simulink model "ATRIAS_vnmc"  (R2015a)
settings: Solver=ode45  StartTime=0.0  StopTime=60  FixedStep=1e-3  MinStep=1e-6  RelTol=1e-3  AbsTol=1e-4
values from neighbouring files (symbols this model uses):
  initial_boom_yaw = initial_boom_yaw + delta_yaw0    [run_model.m]
  max_floor_diff = cost_fun_opts.max_floor_diff    [opt_cmaes.m]    (also in run_model.m; set_all_params_simple.m = 0)
  noise_on_off = cost_fun_opts.noise_on_off    [opt_cmaes.m]    (also in run_model.m; set_all_params_simple.m = 0)
  noise_seed = cost_fun_opts.noise_seed    [opt_cmaes.m]    (also in run_model.m; set_all_params_simple.m = 1)
  noise_variance = cost_fun_opts.noise_variance    [opt_cmaes.m]    (also in run_model.m; set_all_params_simple.m = 0.000174532925199)
  SEA_swing_ctrl_on_off = cost_fun_opts.SEA_swing_ctrl_on_off    [opt_cmaes.m]    (also in run_model.m; set_all_params_simple.m = 0)
  sim_t = simout.twalk    [run_model.m]
  steady_dist = cost_fun_opts.steady_dist    [opt_cmaes.m]    (also in run_model.m; set_all_params_simple.m = 10)
  ts_anim = 0.0333    [run_model.m]
undefined symbols (not defined in the file or in its folder): A1_notch_f1, A2_notch_f1, A_lpf_dtau, A_lpf_velocity, B1_lpf_dtau, B1_lpf_velocity, B1_notch_f1, B2_lpf_dtau, B2_lpf_velocity, B2_notch_f1, b_hmotor, b_leg_spring, b_rotor, base_color_d, boom_color_d, boom_mount_to_center_diagonal, breakaway_friction, c, c_jointstop, com_height_offset, contactThr, coulomb_friction, CtrlPar_theta0, D12_S, D12_T, d_com, ddx_max, ddy_max, delta_phi_max, delta_phi_max_buffer, delta_phi_max_dropoff, delta_phi_min, des_forward_velocity, DS_width, dtau_des_max, dtheta0_vmc, dx0_vmc, dy_max, eref, fblink_color_d, fcut_acceleration, floor_color_d, floor_tile_width, floor_zero_height, FmaxBFSH, FmaxGLU, FmaxHAM, FmaxHFL, FmaxRF, FmaxVAS, FPCtrlPar, friction_linear_zone, g, gain_nodes_sea_torque, gamma_stance_thr, gamma_swing_thr, hip_height, HIP_MTR_MAX_CONT_TORQUE, HIP_MTR_MAX_TORQUE, hshaft_color_d ... (+236)
libraries: sm_lib x280, nesl_utility x174, simulink x114, simulink_extras x58, fl_lib x16, mblibv1 x2, dspswit3 x2
(part 12 of 23)

== system ATRIAS_vnmc/atrias_system/Ground Contact/R Contact/3D Contact ==
  RefPt [m m m] : Inport
  nVec [m m m] : Inport  Port=2
  pVec [m m m] : Inport  Port=3
  vVec [m/s m/s m/s] : Inport  Port=4
  Contact! : EnablePort  StatesWhenEnabling=reset
  Friction Switch : Subsystem
  Kinetic Friction Model : Subsystem
  Logical Operator : Logic  Operator=NOT  AllPortsSameDT=off  OutDataTypeStr=boolean
  Static Friction Model : Subsystem
  Sum : Sum
  Sum1 : Sum
  FnVec [N N N] : Outport  OutputWhenDisabled=reset  InitialOutput=[0 0 0]
      settings: AttributesFormatString=when disabled: %<OutputWhenDisabled>
  FtVec [N N N] : Outport  Port=2  OutputWhenDisabled=reset  InitialOutput=[0 0 0]
      settings: AttributesFormatString=when disabled: %<OutputWhenDisabled>
  wires:
  pVec [m m m]/1 -> Static Friction Model/1(pos [m]), Kinetic Friction Model/2(pos [m m m])
  vVec [m/s m/s m/s]/1 -> Kinetic Friction Model/1(vel [m/s m/s m/s]), Static Friction Model/2(vel [m/s m/s m/s])
  Kinetic Friction Model/2(posFP [m m m]) -> Static Friction Model/4(posFP [m])
  Friction Switch/1(Stiction) -> Static Friction Model/Enable, Logical Operator/1
  Logical Operator/1 -> Kinetic Friction Model/Enable
  nVec [m m m]/1 -> Kinetic Friction Model/4(nVec [m m m])
  Kinetic Friction Model/4(Stiction!) -> Friction Switch/2(Stick!)
  Static Friction Model/1(F_n Stick [N N N]) -> Sum1/1
  Kinetic Friction Model/6(F_n Slide [N N N]) -> Sum1/2
  Kinetic Friction Model/5(F_t Slide [N N N]) -> Sum/2
  Static Friction Model/2(F_t Stick [N N N]) -> Sum/1
  Sum1/1 -> FnVec [N N N]/1  "F_nVec"
  Sum/1 -> FtVec [N N N]/1  "F_tVec"
  Static Friction Model/3(Sliding!) -> Friction Switch/1(Slide!)
  RefPt [m m m]/1 -> Kinetic Friction Model/3(RefPt [m m m])
  Kinetic Friction Model/3(nVec FP [m m m]) -> Static Friction Model/5(nVecFP [m m m])
  Kinetic Friction Model/1(RefPtFP [m m m]) -> Static Friction Model/3(RefPtFP [m m m])

== system ATRIAS_vnmc/atrias_system/Ground Contact/roundTrack (LFoot)/track yaw ==
  xz : Inport
  Abs : Abs
  Compare To Constant : simulink/Logic and Bit Operations/Compare To Constant  relop=>  const=pi  OutDataTypeStr=boolean
  Gain : Gain  Gain=180/pi
  Gain1 : Gain  Gain=180/pi
  Gain2 : Gain  Gain=180/pi
  Memory : Memory
  Scope : Scope  NumInputPorts=4
      settings: YMin=-5~-5~-5~-5  YMax=5~5~5~5
  Sign : Signum
  Sum1 : Sum  Inputs=++|
  Sum2 : Sum  Inputs=|-+
  n*2*pi : Subsystem  TreatAsAtomicUnit=on
  "xz_to_yaw ([0, 2*pi])" : Fcn  Expr=atan2(u(1),-u(2)) +2*pi*(atan2(u(1),-u(2))<0)
  yaw : Outport
  wires:
  Sign/1 -> n*2*pi/2(sign)
  xz/1 -> "xz_to_yaw ([0, 2*pi])"/1
  "xz_to_yaw ([0, 2*pi])"/1 -> Memory/1, Gain1/1, Sum1/2, Sum2/2
  n*2*pi/1(n*2*pi) -> Gain/1, n*2*pi/1((n-1)*2*pi), Sum1/1
  Sum2/1 -> Sign/1, Abs/1
  Abs/1 -> Gain2/1, Compare To Constant/1
  Memory/1 -> Sum2/1
  Compare To Constant/1 -> Scope/3, n*2*pi/Trigger
  Sum1/1 -> yaw/1
  Gain/1 -> Scope/1
  Gain1/1 -> Scope/2
  Gain2/1 -> Scope/4

== system ATRIAS_vnmc/atrias_system/Ground Contact/roundTrack (RFoot)/track yaw ==
  xz : Inport
  Abs : Abs
  Compare To Constant : simulink/Logic and Bit Operations/Compare To Constant  relop=>  const=pi  OutDataTypeStr=boolean
  Gain : Gain  Gain=180/pi
  Gain1 : Gain  Gain=180/pi
  Gain2 : Gain  Gain=180/pi
  Memory : Memory
  Scope : Scope  NumInputPorts=4
      settings: YMin=-5~-5~-5~-5  YMax=5~5~5~5
  Sign : Signum
  Sum1 : Sum  Inputs=++|
  Sum2 : Sum  Inputs=|-+
  n*2*pi : Subsystem  TreatAsAtomicUnit=on
  "xz_to_yaw ([0, 2*pi])" : Fcn  Expr=atan2(u(1),-u(2)) +2*pi*(atan2(u(1),-u(2))<0)
  yaw : Outport
  wires:
  Sign/1 -> n*2*pi/2(sign)
  xz/1 -> "xz_to_yaw ([0, 2*pi])"/1
  "xz_to_yaw ([0, 2*pi])"/1 -> Memory/1, Gain1/1, Sum1/2, Sum2/2
  n*2*pi/1(n*2*pi) -> Gain/1, n*2*pi/1((n-1)*2*pi), Sum1/1
  Sum2/1 -> Sign/1, Abs/1
  Abs/1 -> Gain2/1, Compare To Constant/1
  Memory/1 -> Sum2/1
  Compare To Constant/1 -> Scope/3, n*2*pi/Trigger
  Sum1/1 -> yaw/1
  Gain/1 -> Scope/1
  Gain1/1 -> Scope/2
  Gain2/1 -> Scope/4

== system ATRIAS_vnmc/control/Add Limit Avoidance PD Torques/mechanical limit avoidance/PD Joint Limit ==
  L Scale desired torque : Subsystem
  L mechanical Limit Avoidance Torques (Virtual) : Subsystem
  Mux : Mux
  Mux1 : Mux
  R Mechanical Limit Avoidance Torques (Virtual)1 : Subsystem
  R Scale desired torque : Subsystem
  tau_pd [Nm]x4 : Outport
  des_trq_scale x4 : Outport  Port=2
  tag scope: L_scale_back=global, L_scale_front=global, Ltau_pd_back=global, Ltau_pd_front=global, R_scale_back=global, R_scale_front=global, Rtau_pd_back=global, Rtau_pd_front=global
  wires:
  [Lphi_thigh] -> L mechanical Limit Avoidance Torques (Virtual)/1(phi_thigh [rad])
  [Lphi_shin] -> L mechanical Limit Avoidance Torques (Virtual)/2(phi_shin [rad])
  [Ldphi_thigh] -> L mechanical Limit Avoidance Torques (Virtual)/3(dphi_thigh [rad/s])
  [Ldphi_shin] -> L mechanical Limit Avoidance Torques (Virtual)/4(dphi_shin [rad/s])
  [Rphi_thigh] -> R Mechanical Limit Avoidance Torques (Virtual)1/1(phi_thigh [rad])
  [Rphi_shin] -> R Mechanical Limit Avoidance Torques (Virtual)1/2(phi_shin [rad])
  [Rdphi_thigh] -> R Mechanical Limit Avoidance Torques (Virtual)1/3(dphi_thigh [rad/s])
  [Rdphi_shin] -> R Mechanical Limit Avoidance Torques (Virtual)1/4(dphi_shin [rad/s])
  [Ltau_pd_front] -> Mux/4
  [Ltau_pd_back] -> Mux/3
  [Rtau_pd_front] -> Mux/2
  [Rtau_pd_back] -> Mux/1
  Mux/1 -> tau_pd [Nm]x4/1
  [Rphi_thigh] -> R Scale desired torque/1(phi_thigh [rad])
  [Rphi_shin] -> R Scale desired torque/2(phi_shin [rad])
  [Lphi_thigh] -> L Scale desired torque/1(phi_thigh [rad])
  [Lphi_shin] -> L Scale desired torque/2(phi_shin [rad])
  [L_scale_front] -> Mux1/4
  [L_scale_back] -> Mux1/3
  [R_scale_front] -> Mux1/2
  [R_scale_back] -> Mux1/1
  Mux1/1 -> des_trq_scale x4/1
  R Scale desired torque/1(scale_back) -> [R_scale_back]
  R Scale desired torque/2(scale_front) -> [R_scale_front]
  L Scale desired torque/1(scale_back) -> [L_scale_back]
  L Scale desired torque/2(scale_front) -> [L_scale_front]
  R Mechanical Limit Avoidance Torques (Virtual)1/1(tau_pd_back [Nm]) -> [Rtau_pd_back]
  R Mechanical Limit Avoidance Torques (Virtual)1/2(tau_pd_front [Nm]) -> [Rtau_pd_front]
  L mechanical Limit Avoidance Torques (Virtual)/1(tau_pd_back [Nm]) -> [Ltau_pd_back]
  L mechanical Limit Avoidance Torques (Virtual)/2(tau_pd_front [Nm]) -> [Ltau_pd_front]

== system ATRIAS_vnmc/control/Export Results/track yaw/n*2*pi ==
  (n-1)*2*pi : Inport  LatchByDelayingOutsideSignal=on
  sign : Inport  Port=2
  Trigger : TriggerPort  ZeroCross=off
  Constant : Constant  Value=2*pi
  Gain2 : Gain  Gain=-1
  Product : Product
  Sum : Sum  Inputs=|++
  n*2*pi : Outport  InitialOutput=0
  wires:
  (n-1)*2*pi/1 -> Sum/1
  sign/1 -> Gain2/1
  Gain2/1 -> Product/2
  Constant/1 -> Product/1
  Product/1 -> Sum/2
  Sum/1 -> n*2*pi/1

== system ATRIAS_vnmc/control/Monitor Simulation/Check Ground Penetration/track yaw ==
  xz : Inport
  Abs : Abs
  Compare To Constant : simulink/Logic and Bit Operations/Compare To Constant  relop=>  const=pi  OutDataTypeStr=boolean
  Gain : Gain  Gain=180/pi
  Gain1 : Gain  Gain=180/pi
  Gain2 : Gain  Gain=180/pi
  Memory : Memory
  Scope : Scope  NumInputPorts=4
      settings: YMin=-5~-5~-5~-5  YMax=5~5~5~5
  Sign : Signum
  Sum1 : Sum  Inputs=++|
  Sum2 : Sum  Inputs=|-+
  n*2*pi : Subsystem  TreatAsAtomicUnit=on
  "xz_to_yaw ([0, 2*pi])" : Fcn  Expr=atan2(u(1),-u(2)) +2*pi*(atan2(u(1),-u(2))<0)
  yaw : Outport
  wires:
  Sign/1 -> n*2*pi/2(sign)
  xz/1 -> "xz_to_yaw ([0, 2*pi])"/1
  "xz_to_yaw ([0, 2*pi])"/1 -> Memory/1, Gain1/1, Sum1/2, Sum2/2
  n*2*pi/1(n*2*pi) -> Gain/1, n*2*pi/1((n-1)*2*pi), Sum1/1
  Sum2/1 -> Sign/1, Abs/1
  Abs/1 -> Gain2/1, Compare To Constant/1
  Memory/1 -> Sum2/1
  Compare To Constant/1 -> Scope/3, n*2*pi/Trigger
  Sum1/1 -> yaw/1
  Gain/1 -> Scope/1
  Gain1/1 -> Scope/2
  Gain2/1 -> Scope/4

== system ATRIAS_vnmc/control/Monitor Simulation/Check Ground Penetration1/track yaw ==
  xz : Inport
  Abs : Abs
  Compare To Constant : simulink/Logic and Bit Operations/Compare To Constant  relop=>  const=pi  OutDataTypeStr=boolean
  Gain : Gain  Gain=180/pi
  Gain1 : Gain  Gain=180/pi
  Gain2 : Gain  Gain=180/pi
  Memory : Memory
  Scope : Scope  NumInputPorts=4
      settings: YMin=-5~-5~-5~-5  YMax=5~5~5~5
  Sign : Signum
  Sum1 : Sum  Inputs=++|
  Sum2 : Sum  Inputs=|-+
  n*2*pi : Subsystem  TreatAsAtomicUnit=on
  "xz_to_yaw ([0, 2*pi])" : Fcn  Expr=atan2(u(1),-u(2)) +2*pi*(atan2(u(1),-u(2))<0)
  yaw : Outport
  wires:
  Sign/1 -> n*2*pi/2(sign)
  xz/1 -> "xz_to_yaw ([0, 2*pi])"/1
  "xz_to_yaw ([0, 2*pi])"/1 -> Memory/1, Gain1/1, Sum1/2, Sum2/2
  n*2*pi/1(n*2*pi) -> Gain/1, n*2*pi/1((n-1)*2*pi), Sum1/1
  Sum2/1 -> Sign/1, Abs/1
  Abs/1 -> Gain2/1, Compare To Constant/1
  Memory/1 -> Sum2/1
  Compare To Constant/1 -> Scope/3, n*2*pi/Trigger
  Sum1/1 -> yaw/1
  Gain/1 -> Scope/1
  Gain1/1 -> Scope/2
  Gain2/1 -> Scope/4

== system ATRIAS_vnmc/control/Monitor Simulation/Check Ground Penetration2/track yaw ==
  xz : Inport
  Abs : Abs
  Compare To Constant : simulink/Logic and Bit Operations/Compare To Constant  relop=>  const=pi  OutDataTypeStr=boolean
  Gain : Gain  Gain=180/pi
  Gain1 : Gain  Gain=180/pi
  Gain2 : Gain  Gain=180/pi
  Memory : Memory
  Scope : Scope  NumInputPorts=4
      settings: YMin=-5~-5~-5~-5  YMax=5~5~5~5
  Sign : Signum
  Sum1 : Sum  Inputs=++|
  Sum2 : Sum  Inputs=|-+
  n*2*pi : Subsystem  TreatAsAtomicUnit=on
  "xz_to_yaw ([0, 2*pi])" : Fcn  Expr=atan2(u(1),-u(2)) +2*pi*(atan2(u(1),-u(2))<0)
  yaw : Outport
  wires:
  Sign/1 -> n*2*pi/2(sign)
  xz/1 -> "xz_to_yaw ([0, 2*pi])"/1
  "xz_to_yaw ([0, 2*pi])"/1 -> Memory/1, Gain1/1, Sum1/2, Sum2/2
  n*2*pi/1(n*2*pi) -> Gain/1, n*2*pi/1((n-1)*2*pi), Sum1/1
  Sum2/1 -> Sign/1, Abs/1
  Abs/1 -> Gain2/1, Compare To Constant/1
  Memory/1 -> Sum2/1
  Compare To Constant/1 -> Scope/3, n*2*pi/Trigger
  Sum1/1 -> yaw/1
  Gain/1 -> Scope/1
  Gain1/1 -> Scope/2
  Gain2/1 -> Scope/4

== system ATRIAS_vnmc/control/Monitor Simulation/Check Ground Penetration3/track yaw ==
  xz : Inport
  Abs : Abs
  Compare To Constant : simulink/Logic and Bit Operations/Compare To Constant  relop=>  const=pi  OutDataTypeStr=boolean
  Gain : Gain  Gain=180/pi
  Gain1 : Gain  Gain=180/pi
  Gain2 : Gain  Gain=180/pi
  Memory : Memory
  Scope : Scope  NumInputPorts=4
      settings: YMin=-5~-5~-5~-5  YMax=5~5~5~5
  Sign : Signum
  Sum1 : Sum  Inputs=++|
  Sum2 : Sum  Inputs=|-+
  n*2*pi : Subsystem  TreatAsAtomicUnit=on
  "xz_to_yaw ([0, 2*pi])" : Fcn  Expr=atan2(u(1),-u(2)) +2*pi*(atan2(u(1),-u(2))<0)
  yaw : Outport
  wires:
  Sign/1 -> n*2*pi/2(sign)
  xz/1 -> "xz_to_yaw ([0, 2*pi])"/1
  "xz_to_yaw ([0, 2*pi])"/1 -> Memory/1, Gain1/1, Sum1/2, Sum2/2
  n*2*pi/1(n*2*pi) -> Gain/1, n*2*pi/1((n-1)*2*pi), Sum1/1
  Sum2/1 -> Sign/1, Abs/1
  Abs/1 -> Gain2/1, Compare To Constant/1
  Memory/1 -> Sum2/1
  Compare To Constant/1 -> Scope/3, n*2*pi/Trigger
  Sum1/1 -> yaw/1
  Gain/1 -> Scope/1
  Gain1/1 -> Scope/2
  Gain2/1 -> Scope/4

== system ATRIAS_vnmc/control/Monitor Simulation/Step Length History/Measure Step Length ==
  x_heelstrike_prev [m] : Inport
  x_heelstrike [m] : Inport  Port=2
  Trigger : TriggerPort
  Sum : Sum  Inputs=|-+
  Step Length [m] : Outport  InitialOutput=0
  wires:
  x_heelstrike_prev [m]/1 -> Sum/1
  x_heelstrike [m]/1 -> Sum/2
  Sum/1 -> Step Length [m]/1

== system ATRIAS_vnmc/control/Monitor Simulation/Step Length History/Queue1 ==
  footStrike [1/0] : Inport
  stepLength0 [m] : Inport  Port=2
  Memory{2..7} (6 alike) : Memory
  Vector Concatenate : Concatenate  NumInputs=7
  cascade : Subsystem  TreatAsAtomicUnit=on
  cascade1 : Subsystem  TreatAsAtomicUnit=on
  cascade2 : Subsystem  TreatAsAtomicUnit=on
  cascade3 : Subsystem  TreatAsAtomicUnit=on
  cascade4 : Subsystem  TreatAsAtomicUnit=on
  cascade5 : Subsystem  TreatAsAtomicUnit=on
  footLengthHist [m,m,m,m,m,m,m] : Outport
  wires:
  Memory2/1 -> cascade/1(In1)
  Memory3/1 -> cascade1/1(In1)
  Memory4/1 -> cascade2/1(In1)
  cascade1/1(Out1) -> Memory4/1, Vector Concatenate/3
  Memory5/1 -> cascade3/1(In1)
  cascade/1(Out1) -> Vector Concatenate/2, Memory3/1
  Memory6/1 -> cascade4/1(In1)
  cascade3/1(Out1) -> Memory6/1, Vector Concatenate/5
  cascade4/1(Out1) -> Vector Concatenate/6, Memory7/1
  Memory7/1 -> cascade5/1(In1)
  cascade2/1(Out1) -> Vector Concatenate/4, Memory5/1
  cascade5/1(Out1) -> Vector Concatenate/7
  Vector Concatenate/1 -> footLengthHist [m,m,m,m,m,m,m]/1
  [footStrike] -> cascade/Trigger
  [footStrike] -> cascade3/Trigger
  [footStrike] -> cascade5/Trigger
  [footStrike] -> cascade4/Trigger
  stepLength0 [m]/1 -> Vector Concatenate/1, Memory2/1
  [footStrike] -> cascade1/Trigger
  [footStrike] -> cascade2/Trigger
  footStrike [1/0]/1 -> [footStrike]

== system ATRIAS_vnmc/control/Monitor Simulation/Step Length History/x_footstrike ==
  Footstrike [1/0] : Inport
  x_LFoot [m] : Inport  Port=2
  LHeel Contact [1/0] : Inport  Port=3
  RHeel Contact [1/0] : Inport  Port=4
  x_RFoot [m] : Inport  Port=5
  Data Type Conversion : DataTypeConversion  OutDataTypeStr=double
  Data Type Conversion1 : DataTypeConversion  OutDataTypeStr=double
  Detect Increase2 : simulink/Logic and Bit Operations/Detect Increase  vinit=0.0  InputProcessing=Inherited  OutDataTypeStr=boolean
  Detect Increase3 : simulink/Logic and Bit Operations/Detect Increase  vinit=0.0  InputProcessing=Inherited  OutDataTypeStr=boolean
  Product2 : Product
  Product3 : Product
  S-R Flip-Flop : simulink_extras/Flip Flops/S-R Flip-Flop  initial_condition=0
  Sum4 : Sum
  Triggered Subsystem : Subsystem  TreatAsAtomicUnit=on
  x_footstrike [m] : Outport
  wires:
  LHeel Contact [1/0]/1 -> Detect Increase2/1
  RHeel Contact [1/0]/1 -> Detect Increase3/1
  Detect Increase2/1 -> S-R Flip-Flop/1
  Detect Increase3/1 -> S-R Flip-Flop/2
  S-R Flip-Flop/1 -> Data Type Conversion/1
  Data Type Conversion/1 -> Product2/2
  x_LFoot [m]/1 -> Product2/1
  Data Type Conversion1/1 -> Product3/1
  x_RFoot [m]/1 -> Product3/2
  S-R Flip-Flop/2 -> Data Type Conversion1/1
  Product2/1 -> Sum4/1
  Product3/1 -> Sum4/2
  Sum4/1 -> Triggered Subsystem/1(x)  "x_touchdown"
  Footstrike [1/0]/1 -> Triggered Subsystem/Trigger
  Triggered Subsystem/1(x_hold) -> x_footstrike [m]/1

== system ATRIAS_vnmc/control/Plot Signals/VMC Plots/Measure COM Acc ==
  Constant12 : Constant  Value=l_boom
  Constant14 : Constant  Value=boom_mount_to_center_diagonal
  Constant6 : Constant  Value=boom_mount_to_center_diagonal
  Constant7 : Constant  Value=l_boom
  Constant8 : Constant  Value=boom_mount_to_center_diagonal
  Constant9 : Constant  Value=l_boom
  Derivative : Derivative  CoefficientInTFapproximation=100
  Derivative1 : Derivative  CoefficientInTFapproximation=100
  Gain : Gain  Gain=-1
  Product2 : Product  Inputs=3
  Product3 : Product  Inputs=4
  Product5 : Product  Inputs=3
  Sum{3..5,8} (4 alike) : Sum  Inputs=|++
  Trigonometric Function1 : Trigonometry  Operator=cos
  Trigonometric Function2 : Trigonometry
  Trigonometric Function4 : Trigonometry  Operator=cos
  tag scope: ddtheta_com_cont=global, ddx_com_cont=global, ddy_com_cont=global, dtheta_com_cont=global, dx_com_cont=global, dy_com_cont=global
  wires:
  [dq13] -> [dtheta_com_cont]
  [dx_com_cont] -> Derivative/1
  [dq12] -> Product2/1
  Sum3/1 -> Product2/3
  Constant7/1 -> Sum3/1
  Constant6/1 -> Sum3/2
  Trigonometric Function1/1 -> Product2/2
  [q11] -> Trigonometric Function1/1
  Product2/1 -> Sum4/1  "x"
  [q12] -> Product3/3
  Sum5/1 -> Product3/4
  Constant9/1 -> Sum5/1
  Constant8/1 -> Sum5/2
  Trigonometric Function2/1 -> Gain/1
  [q11] -> Trigonometric Function2/1
  Product3/1 -> Sum4/2
  Gain/1 -> Product3/2
  [dq11] -> Product3/1
  Sum4/1 -> [dx_com_cont]
  Sum8/1 -> Product5/3
  Constant12/1 -> Sum8/1
  Constant14/1 -> Sum8/2
  Trigonometric Function4/1 -> Product5/2
  [q11] -> Trigonometric Function4/1
  Product5/1 -> [dy_com_cont]
  [dq11] -> Product5/1
  [dy_com_cont] -> Derivative1/1
  [ddq13] -> [ddtheta_com_cont]
  Derivative/1 -> [ddx_com_cont]
  Derivative1/1 -> [ddy_com_cont]

== system ATRIAS_vnmc/control/SEA Ctrl/SEA Controller (Torque)/Antiresonance Compensation ==
  Torque : Inport
  Notch Filter (Flight) : DiscreteTransferFcn  Numerator=[K_notch_f1 K_notch_f1*A1_notch_f1 K_notch_f1*A2_notch_f1]  Denominator=[1 B1_notch_f1 B2_notch_f1]  SampleTime=sample_time
  Filtered Torque : Outport
  wires:
  Notch Filter (Flight)/1 -> Filtered Torque/1
  Torque/1 -> Notch Filter (Flight)/1

== system ATRIAS_vnmc/control/SEA Ctrl/SEA Controller (Torque)/Friction Compensation ==
  Motor Velocity [rad/s] : Inport
  Gain2 : Gain  Gain=sea_coulomb_friction_direction_switch_sensitivity
  KdGain2 : Gain  Description=xPCTag(1)=kd_sea_torque;  Gain=sea_coulomb_friction
  Trigonometric Function : Trigonometry  Operator=tanh
  Friction Compensation [Nm] : Outport
  wires:
  Trigonometric Function/1 -> KdGain2/1
  Gain2/1 -> Trigonometric Function/1
  Motor Velocity [rad/s]/1 -> Gain2/1
  KdGain2/1 -> Friction Compensation [Nm]/1

== system ATRIAS_vnmc/control/SEA Ctrl/SEA Controller (Torque)/Loaded Unloaded Switch ==
  Loaded Signal : Inport
  Unloaded Signal : Inport  Port=2
  Loaded/Unloaded [1/0] x4 : Inport  Port=3
  Demux : Demux
  Demux1 : Demux
  Demux2 : Demux
  Mux : Mux
  Switch{,1..3} (4 alike) : Switch  Criteria=u2 ~= 0
  Signal : Outport
  wires:
  Demux2/1 -> Switch/3
  Demux2/2 -> Switch1/3
  Demux2/3 -> Switch2/3
  Demux2/4 -> Switch3/3
  Unloaded Signal/1 -> Demux2/1
  Demux1/4 -> Switch3/1
  Demux1/3 -> Switch2/1
  Demux1/2 -> Switch1/1
  Demux1/1 -> Switch/1
  Loaded Signal/1 -> Demux1/1
  Demux/1 -> Switch/2
  Switch/1 -> Mux/1
  Mux/1 -> Signal/1
  Loaded/Unloaded [1/0] x4/1 -> Demux/1
  Switch3/1 -> Mux/4
  Switch2/1 -> Mux/3
  Switch1/1 -> Mux/2
  Demux/2 -> Switch1/2
  Demux/3 -> Switch2/2
  Demux/4 -> Switch3/2

== system ATRIAS_vnmc/control/SEA Ctrl/SEA Controller (Torque)/filtered_derivative ==
  x : Inport
  Low Pass Discrete Derivative : Subsystem
  dx/dt : Outport
  wires:
  x/1 -> Low Pass Discrete Derivative/1(q)
  Low Pass Discrete Derivative/1(dq) -> dx/dt/1

== system ATRIAS_vnmc/control/Virtual Model Control/COM PD Law/Hold Values ==
  in : Inport
  Trigger : TriggerPort  ShowOutputPort=on  PortDimensions=1
  Subsystem : Subsystem
  out : Outport
  wires:
  in/1 -> Subsystem/1(in)
  Subsystem/1(out) -> out/1
  Trigger/1 -> Subsystem/Enable

== system ATRIAS_vnmc/control/Virtual Model Control/COM PD Law/Hold Values1 ==
  in : Inport
  Trigger : TriggerPort  ShowOutputPort=on  PortDimensions=1
  Subsystem : Subsystem
  out : Outport
  wires:
  in/1 -> Subsystem/1(in)
  Subsystem/1(out) -> out/1
  Trigger/1 -> Subsystem/Enable

== system ATRIAS_vnmc/control/Virtual Model Control/Flight PD/Back//Front Motor PD1 ==
  Desired Position [rad] [back front] : Inport
  Desired Velocity [rad/s] [back front] : Inport  Port=2
  Desired Acceleration [rad/s^2] [back front] : Inport  Port=3
  Measured Position [rad] [back front] : Inport  Port=4
  Measured Velocity [rad/s] [back front] : Inport  Port=5
  Product : Product
  Sum1 : Sum  Inputs=|++
  Sum7 : Sum  Inputs=|+-
  Sum8 : Sum  Inputs=|+-
  Sum9 : Sum
  kd : Gain  Gain=kd_motor
  kp : Gain  Gain=kp_motor
  reflected inertia : Constant  Value=j_motor
  Commanded Torque [Nm] [back front] : Outport
  wires:
  kp/1 -> Sum9/1
  Sum7/1 -> kp/1
  Measured Position [rad] [back front]/1 -> Sum7/2
  Sum9/1 -> Sum1/1
  Sum8/1 -> kd/1
  Desired Position [rad] [back front]/1 -> Sum7/1
  kd/1 -> Sum9/2
  Measured Velocity [rad/s] [back front]/1 -> Sum8/2
  Desired Acceleration [rad/s^2] [back front]/1 -> Product/1
  Product/1 -> Sum1/2
  Sum1/1 -> Commanded Torque [Nm] [back front]/1
  Desired Velocity [rad/s] [back front]/1 -> Sum8/1
  reflected inertia/1 -> Product/2

== system ATRIAS_vnmc/control/Virtual Model Control/Flight PD/Back//Front Motor PD2 ==
  Desired Position [rad] [back front] : Inport
  Desired Velocity [rad/s] [back front] : Inport  Port=2
  Desired Acceleration [rad/s^2] [back front] : Inport  Port=3
  Measured Position [rad] [back front] : Inport  Port=4
  Measured Velocity [rad/s] [back front] : Inport  Port=5
  Product : Product
  Sum1 : Sum  Inputs=|++
  Sum7 : Sum  Inputs=|+-
  Sum8 : Sum  Inputs=|+-
  Sum9 : Sum
  kd : Gain  Gain=kd_motor
  kp : Gain  Gain=kp_motor
  reflected inertia : Constant  Value=j_motor
  Commanded Torque [Nm] [back front] : Outport
  wires:
  kp/1 -> Sum9/1
  Sum7/1 -> kp/1
  Measured Position [rad] [back front]/1 -> Sum7/2
  Sum9/1 -> Sum1/1
  Sum8/1 -> kd/1
  Desired Position [rad] [back front]/1 -> Sum7/1
  kd/1 -> Sum9/2
  Measured Velocity [rad/s] [back front]/1 -> Sum8/2
  Desired Acceleration [rad/s^2] [back front]/1 -> Product/1
  Product/1 -> Sum1/2
  Sum1/1 -> Commanded Torque [Nm] [back front]/1
  Desired Velocity [rad/s] [back front]/1 -> Sum8/1
  reflected inertia/1 -> Product/2

== system ATRIAS_vnmc/control/Virtual Model Control/Swing Leg Behavior1/Back//Front Motor PD ==
  Desired Position [rad] [back front] : Inport
  Desired Velocity [rad/s] [back front] : Inport  Port=2
  Desired Acceleration [rad/s^2] [back front] : Inport  Port=3
  Measured Position [rad] [back front] : Inport  Port=4
  Measured Velocity [rad/s] [back front] : Inport  Port=5
  Product : Product
  Sum1 : Sum  Inputs=|++
  Sum7 : Sum  Inputs=|+-
  Sum8 : Sum  Inputs=|+-
  Sum9 : Sum
  kd : Gain  Gain=kd_motor
  kp : Gain  Gain=kp_motor
  reflected inertia : Constant  Value=j_motor
  Commanded Torque [Nm] [back front] : Outport
  wires:
  reflected inertia/1 -> Product/2
  Desired Velocity [rad/s] [back front]/1 -> Sum8/1
  Sum1/1 -> Commanded Torque [Nm] [back front]/1
  Product/1 -> Sum1/2
  Desired Acceleration [rad/s^2] [back front]/1 -> Product/1
  Measured Velocity [rad/s] [back front]/1 -> Sum8/2
  kd/1 -> Sum9/2
  Desired Position [rad] [back front]/1 -> Sum7/1
  Sum8/1 -> kd/1
  Sum9/1 -> Sum1/1
  Measured Position [rad] [back front]/1 -> Sum7/2
  Sum7/1 -> kp/1
  kp/1 -> Sum9/1

== system ATRIAS_vnmc/control/Virtual Model Control/Swing Leg Behavior1/Hold Values ==
  in : Inport
  Trigger : TriggerPort  ShowOutputPort=on  PortDimensions=1
  Subsystem : Subsystem
  out : Outport
  wires:
  Trigger/1 -> Subsystem/Enable
  Subsystem/1(out) -> out/1
  in/1 -> Subsystem/1(in)

== system ATRIAS_vnmc/control/Virtual Model Control/Swing Leg Behavior1/Hold Values1 ==
  in : Inport
  Trigger : TriggerPort  ShowOutputPort=on  PortDimensions=1
  Subsystem : Subsystem
  out : Outport
  wires:
  Trigger/1 -> Subsystem/Enable
  Subsystem/1(out) -> out/1
  in/1 -> Subsystem/1(in)

== system ATRIAS_vnmc/control/Virtual Model Control/Swing Leg Behavior2/Back//Front Motor PD ==
  Desired Position [rad] [back front] : Inport
  Desired Velocity [rad/s] [back front] : Inport  Port=2
  Desired Acceleration [rad/s^2] [back front] : Inport  Port=3
  Measured Position [rad] [back front] : Inport  Port=4
  Measured Velocity [rad/s] [back front] : Inport  Port=5
  Product : Product
  Sum1 : Sum  Inputs=|++
  Sum7 : Sum  Inputs=|+-
  Sum8 : Sum  Inputs=|+-
  Sum9 : Sum
  kd : Gain  Gain=kd_motor
  kp : Gain  Gain=kp_motor
  reflected inertia : Constant  Value=j_motor
  Commanded Torque [Nm] [back front] : Outport
  wires:
  kp/1 -> Sum9/1
  Sum7/1 -> kp/1
  Measured Position [rad] [back front]/1 -> Sum7/2
  Sum9/1 -> Sum1/1
  Sum8/1 -> kd/1
  Desired Position [rad] [back front]/1 -> Sum7/1
  kd/1 -> Sum9/2
  Measured Velocity [rad/s] [back front]/1 -> Sum8/2
  Desired Acceleration [rad/s^2] [back front]/1 -> Product/1
  Product/1 -> Sum1/2
  Sum1/1 -> Commanded Torque [Nm] [back front]/1
  Desired Velocity [rad/s] [back front]/1 -> Sum8/1
  reflected inertia/1 -> Product/2

== system ATRIAS_vnmc/control/Virtual Model Control/Swing Leg Behavior2/Hold Values ==
  in : Inport
  Trigger : TriggerPort  ShowOutputPort=on  PortDimensions=1
  Subsystem : Subsystem
  out : Outport
  wires:
  in/1 -> Subsystem/1(in)
  Subsystem/1(out) -> out/1
  Trigger/1 -> Subsystem/Enable

== system ATRIAS_vnmc/control/Virtual Model Control/Swing Leg Behavior2/Hold Values1 ==
  in : Inport
  Trigger : TriggerPort  ShowOutputPort=on  PortDimensions=1
  Subsystem : Subsystem
  out : Outport
  wires:
  in/1 -> Subsystem/1(in)
  Subsystem/1(out) -> out/1
  Trigger/1 -> Subsystem/Enable

== system ATRIAS_vnmc/control/Virtual Model Control/Swing Leg Behavior3/Back//Front Motor PD ==
  Desired Position [rad] [back front] : Inport
  Desired Velocity [rad/s] [back front] : Inport  Port=2
  Desired Acceleration [rad/s^2] [back front] : Inport  Port=3
  Measured Position [rad] [back front] : Inport  Port=4
  Measured Velocity [rad/s] [back front] : Inport  Port=5
  Product : Product
  Sum1 : Sum  Inputs=|++
  Sum7 : Sum  Inputs=|+-
  Sum8 : Sum  Inputs=|+-
  Sum9 : Sum
  kd : Gain  Gain=kd_motor
  kp : Gain  Gain=kp_motor
  reflected inertia : Constant  Value=j_motor
  Commanded Torque [Nm] [back front] : Outport
  wires:
  reflected inertia/1 -> Product/2
  Desired Velocity [rad/s] [back front]/1 -> Sum8/1
  Sum1/1 -> Commanded Torque [Nm] [back front]/1
  Product/1 -> Sum1/2
  Desired Acceleration [rad/s^2] [back front]/1 -> Product/1
  Measured Velocity [rad/s] [back front]/1 -> Sum8/2
  kd/1 -> Sum9/2
  Desired Position [rad] [back front]/1 -> Sum7/1
  Sum8/1 -> kd/1
  Sum9/1 -> Sum1/1
  Measured Position [rad] [back front]/1 -> Sum7/2
  Sum7/1 -> kp/1
  kp/1 -> Sum9/1

== system ATRIAS_vnmc/control/Virtual Model Control/Swing Leg Behavior3/Hold Values ==
  in : Inport
  Trigger : TriggerPort  ShowOutputPort=on  PortDimensions=1
  Subsystem : Subsystem
  out : Outport
  wires:
  Trigger/1 -> Subsystem/Enable
  Subsystem/1(out) -> out/1
  in/1 -> Subsystem/1(in)

== system ATRIAS_vnmc/control/Virtual Model Control/Swing Leg Behavior3/Hold Values1 ==
  in : Inport
  Trigger : TriggerPort  ShowOutputPort=on  PortDimensions=1
  Subsystem : Subsystem
  out : Outport
  wires:
  Trigger/1 -> Subsystem/Enable
  Subsystem/1(out) -> out/1
  in/1 -> Subsystem/1(in)

== system ATRIAS_vnmc/control/Virtual Neuromuscular Control/Higher Control Layer/Double Support ==
  LStance : Inport
  RStance : Inport  Port=2
  Lalpha_tgt : Inport  Port=3
  Lphi34 : Inport  Port=4
  Lphi23 : Inport  Port=5
  Ralpha_tgt : Inport  Port=6
  Rphi34 : Inport  Port=7
  Rphi23 : Inport  Port=8
  Abs : Abs  ZeroCross=off
  Abs1 : Abs  ZeroCross=off
  Lalpha' : Fcn  Expr=u(1) - u(2)/2
  Logical Operator1 : Logic  Operator=NOR  AllPortsSameDT=off
  Logical Operator2 : Logic  Operator=NOT  AllPortsSameDT=off
  Logical Operator3 : Logic  AllPortsSameDT=off
  Logical Operator4 : Logic  AllPortsSameDT=off
  Logical Operator5 : Logic  AllPortsSameDT=off
  Mux1 : Mux  Inputs=2
  Mux5 : Mux  Inputs=2
  Ralpha' : Fcn  Expr=u(1) - u(2)/2
  Relational Operator : RelationalOperator  Operator=>  ZeroCross=off
  Sum5 : Sum  Inputs=-+|
  Sum7 : Sum  Inputs=-+|
  RonL : Outport
  Flight : Outport  Port=2
  LonR : Outport  Port=3
  DS : Outport  Port=4
  wires:
  Lalpha'/1 -> Sum7/2  "Lalpha"
  Mux5/1 -> Lalpha'/1
  Ralpha'/1 -> Sum5/2
  Mux1/1 -> Ralpha'/1
  Sum5/1 -> Abs/1
  Sum7/1 -> Abs1/1
  LStance/1 -> Logical Operator3/1, Logical Operator1/1
  RStance/1 -> Logical Operator3/2, Logical Operator1/2
  Lalpha_tgt/1 -> Sum7/1
  Lphi34/1 -> Mux5/1
  Lphi23/1 -> Mux5/2
  Ralpha_tgt/1 -> Sum5/1
  Rphi34/1 -> Mux1/1
  Rphi23/1 -> Mux1/2
  Logical Operator1/1 -> Flight/1
  Abs1/1 -> Relational Operator/1
  Abs/1 -> Relational Operator/2
  Logical Operator4/1 -> RonL/1
  Logical Operator2/1 -> Logical Operator5/2
  Logical Operator5/1 -> LonR/1
  Relational Operator/1 -> Logical Operator2/1, Logical Operator4/2
  Logical Operator3/1 -> Logical Operator5/1, Logical Operator4/1, DS/1

== system ATRIAS_vnmc/control/Virtual Neuromuscular Control/Muscle Layer/GLU ==
  note: SOLEUS Muscle-Tendon Dynamics
  note: Excitation Contraction Coupling
  STIM : Inport
  lmtc [m] : Inport  Port=2
  1 : Product  Inputs=**  SaturateOnIntegerOverflow=on  InputSameDT=on  OutDataTypeStr=Inherit: Same as first input
  1/lslack : Gain  Gain=1/lslackGLU  SaturateOnIntegerOverflow=on  OutDataTypeStr=Inherit: Same as input  ParamDataTypeStr=Inherit: Same as input
  BE force-length relation : Subsystem
  CE force-length relation : Subsystem
  CE inverse force-velocity relation : Subsystem
  Constant : Constant  Value=lslackGLU
  ECC TransferFcn : simulink_extras/Additional Linear/Transfer Fcn (with initial outputs)  N=[1]  D="[tau  1]"  Y0=preA  U0=0
      settings: AttributesFormatString=pre-activation: %<Y0>
  Fmax : Gain  Gain=FmaxGLU  SaturateOnIntegerOverflow=on  OutDataTypeStr=Inherit: Same as input  ParamDataTypeStr=Inherit: Same as input
  Fv = Fse / (A*Fce) : Product  Inputs=*/  SaturateOnIntegerOverflow=on  InputSameDT=on  OutDataTypeStr=Inherit: Same as first input
  Integrator : Integrator  InitialConditionSource=external  LowerSaturationLimit=0.05
  PE force-length relation : Subsystem
  SE force-length relation : Subsystem
  Saturation : Saturate  UpperLimit=1  LowerLimit=0.01
  Sum : Sum  Inputs=|+-  SaturateOnIntegerOverflow=on  InputSameDT=on  OutDataTypeStr=Inherit: Same as first input
  Sum2 : Sum  Inputs=|-+  SaturateOnIntegerOverflow=on  InputSameDT=on  OutDataTypeStr=Inherit: Same as first input
  Sum3 : Sum  SaturateOnIntegerOverflow=on  InputSameDT=on  OutDataTypeStr=Inherit: Same as first input
  Sum4 : Sum  SaturateOnIntegerOverflow=on  InputSameDT=on  OutDataTypeStr=Inherit: Same as first input
  lce/lopt : Gain  Gain=1/loptGLU  SaturateOnIntegerOverflow=on  OutDataTypeStr=Inherit: Same as input  ParamDataTypeStr=Inherit: Same as input
  vmax*lopt : Gain  Gain=vmaxGLU*loptGLU  SaturateOnIntegerOverflow=on  OutDataTypeStr=Inherit: Same as input  ParamDataTypeStr=Inherit: Same as input
  Fmtc : Outport  InitialOutput=0
  Lce : Outport  Port=2  InitialOutput=0
  Vce : Outport  Port=3  InitialOutput=0
  A : Outport  Port=4  InitialOutput=0
  wires:
  Integrator/1 -> Sum/2, lce/lopt/1, Lce/1  "lce"
  Sum/1 -> 1/lslack/1  "lse"
  lce/lopt/1 -> CE force-length relation/1(lce [lopt]), BE force-length relation/1(lce [lopt]), PE force-length relation/1(lce [lopt])
  Fv = Fse / (A*Fce)/1 -> CE inverse force-velocity relation/1(Fv[Fmax])  "fv"
  vmax*lopt/1 -> Integrator/1, Vce/1  "vce"
  lmtc [m]/1 -> Sum2/2, Sum/1  "lmtc"
  Fmax/1 -> Fmtc/1  "Fmtc"
  1/lslack/1 -> SE force-length relation/1(lse [lslack])
  SE force-length relation/1(fse [Fmax]) -> Fmax/1, Sum4/1
  Sum2/1 -> Integrator/2
  Constant/1 -> Sum2/1
  CE force-length relation/1(fce [Fmax]) -> 1/1
  Sum4/1 -> Fv = Fse / (A*Fce)/1
  PE force-length relation/1(fpe [Fmax]) -> Sum3/1
  1/1 -> Sum3/2
  BE force-length relation/1(fbe [Fmax]) -> Sum4/2
  Sum3/1 -> Fv = Fse / (A*Fce)/2
  CE inverse force-velocity relation/1(v[vmax]) -> vmax*lopt/1
  STIM/1 -> ECC TransferFcn/1
  ECC TransferFcn/1 -> Saturation/1
  Saturation/1 -> A/1, 1/2

== system ATRIAS_vnmc/control/Virtual Neuromuscular Control/Muscle Layer/GLU Link ==
  note: GLUTEUS Attachment
  phi34 [rad] : Inport
  Constant : Constant  Value=lslackGLU+loptGLU
  Constant1 : Constant  Value=rGLU
  Constant2 : Constant  Value=phirefGLU
  Gain2 : Gain  Gain=rhoGLU
  Product : Product  RndMeth=Zero
  Sum2 : Sum  Inputs=|+-
  Sum5 : Sum  Inputs=|+-
  lmtu [m] : Outport
  lever [m] : Outport  Port=2
  wires:
  Constant/1 -> Sum5/1
  Sum5/1 -> lmtu [m]/1
  Product/1 -> Gain2/1
  phi34 [rad]/1 -> Sum2/1
  Constant2/1 -> Sum2/2
  Sum2/1 -> Product/1
  Constant1/1 -> Product/2, lever [m]/1
  Gain2/1 -> Sum5/2

== system ATRIAS_vnmc/control/Virtual Neuromuscular Control/Muscle Layer/GLU Link1 ==
  note: GLUTEUS Attachment
  phi34 [rad] : Inport
  Constant : Constant  Value=lslackGLU+loptGLU
  Constant1 : Constant  Value=rGLU
  Constant2 : Constant  Value=phirefGLU
  Gain2 : Gain  Gain=rhoGLU
  Product : Product  RndMeth=Zero
  Sum2 : Sum  Inputs=|+-
  Sum5 : Sum  Inputs=|+-
  lmtu [m] : Outport
  lever [m] : Outport  Port=2
  wires:
  Constant/1 -> Sum5/1
  Sum5/1 -> lmtu [m]/1
  Product/1 -> Gain2/1
  phi34 [rad]/1 -> Sum2/1
  Constant2/1 -> Sum2/2
  Sum2/1 -> Product/1
  Constant1/1 -> Product/2, lever [m]/1
  Gain2/1 -> Sum5/2

== system ATRIAS_vnmc/control/Virtual Neuromuscular Control/Muscle Layer/GLU1 ==
  note: SOLEUS Muscle-Tendon Dynamics
  note: Excitation Contraction Coupling
  STIM : Inport
  lmtc [m] : Inport  Port=2
  1 : Product  Inputs=**  SaturateOnIntegerOverflow=on  InputSameDT=on  OutDataTypeStr=Inherit: Same as first input
  1/lslack : Gain  Gain=1/lslackGLU  SaturateOnIntegerOverflow=on  OutDataTypeStr=Inherit: Same as input  ParamDataTypeStr=Inherit: Same as input
  BE force-length relation : Subsystem
  CE force-length relation : Subsystem
  CE inverse force-velocity relation : Subsystem
  Constant : Constant  Value=lslackGLU
  ECC TransferFcn : simulink_extras/Additional Linear/Transfer Fcn (with initial outputs)  N=[1]  D="[tau  1]"  Y0=preA  U0=0
      settings: AttributesFormatString=pre-activation: %<Y0>
  Fmax : Gain  Gain=FmaxGLU  SaturateOnIntegerOverflow=on  OutDataTypeStr=Inherit: Same as input  ParamDataTypeStr=Inherit: Same as input
  Fv = Fse / (A*Fce) : Product  Inputs=*/  SaturateOnIntegerOverflow=on  InputSameDT=on  OutDataTypeStr=Inherit: Same as first input
  Integrator : Integrator  InitialConditionSource=external  LowerSaturationLimit=0.05
  PE force-length relation : Subsystem
  SE force-length relation : Subsystem
  Saturation : Saturate  UpperLimit=1  LowerLimit=0.01
  Sum : Sum  Inputs=|+-  SaturateOnIntegerOverflow=on  InputSameDT=on  OutDataTypeStr=Inherit: Same as first input
  Sum2 : Sum  Inputs=|-+  SaturateOnIntegerOverflow=on  InputSameDT=on  OutDataTypeStr=Inherit: Same as first input
  Sum3 : Sum  SaturateOnIntegerOverflow=on  InputSameDT=on  OutDataTypeStr=Inherit: Same as first input
  Sum4 : Sum  SaturateOnIntegerOverflow=on  InputSameDT=on  OutDataTypeStr=Inherit: Same as first input
  lce/lopt : Gain  Gain=1/loptGLU  SaturateOnIntegerOverflow=on  OutDataTypeStr=Inherit: Same as input  ParamDataTypeStr=Inherit: Same as input
  vmax*lopt : Gain  Gain=vmaxGLU*loptGLU  SaturateOnIntegerOverflow=on  OutDataTypeStr=Inherit: Same as input  ParamDataTypeStr=Inherit: Same as input
  Fmtc : Outport  InitialOutput=0
  Lce : Outport  Port=2  InitialOutput=0
  Vce : Outport  Port=3  InitialOutput=0
  A : Outport  Port=4  InitialOutput=0
  wires:
  Integrator/1 -> Sum/2, lce/lopt/1, Lce/1  "lce"
  Sum/1 -> 1/lslack/1  "lse"
  lce/lopt/1 -> CE force-length relation/1(lce [lopt]), BE force-length relation/1(lce [lopt]), PE force-length relation/1(lce [lopt])
  Fv = Fse / (A*Fce)/1 -> CE inverse force-velocity relation/1(Fv[Fmax])  "fv"
  vmax*lopt/1 -> Integrator/1, Vce/1  "vce"
  lmtc [m]/1 -> Sum2/2, Sum/1  "lmtc"
  Fmax/1 -> Fmtc/1  "Fmtc"
  1/lslack/1 -> SE force-length relation/1(lse [lslack])
  SE force-length relation/1(fse [Fmax]) -> Fmax/1, Sum4/1
  Sum2/1 -> Integrator/2
  Constant/1 -> Sum2/1
  CE force-length relation/1(fce [Fmax]) -> 1/1
  Sum4/1 -> Fv = Fse / (A*Fce)/1
  PE force-length relation/1(fpe [Fmax]) -> Sum3/1
  1/1 -> Sum3/2
  BE force-length relation/1(fbe [Fmax]) -> Sum4/2
  Sum3/1 -> Fv = Fse / (A*Fce)/2
  CE inverse force-velocity relation/1(v[vmax]) -> vmax*lopt/1
  STIM/1 -> ECC TransferFcn/1
  ECC TransferFcn/1 -> Saturation/1
  Saturation/1 -> A/1, 1/2

== system ATRIAS_vnmc/control/Virtual Neuromuscular Control/Muscle Layer/HAM ==
  note: SOLEUS Muscle-Tendon Dynamics
  note: Excitation Contraction Coupling
  STIM : Inport
  lmtc [m] : Inport  Port=2
  1 : Product  Inputs=**  SaturateOnIntegerOverflow=on  InputSameDT=on  OutDataTypeStr=Inherit: Same as first input
  1/lslack : Gain  Gain=1/lslackHAM  SaturateOnIntegerOverflow=on  OutDataTypeStr=Inherit: Same as input  ParamDataTypeStr=Inherit: Same as input
  BE force-length relation : Subsystem
  CE force-length relation : Subsystem
  CE inverse force-velocity relation : Subsystem
  Constant : Constant  Value=lslackHAM
  ECC TransferFcn : simulink_extras/Additional Linear/Transfer Fcn (with initial outputs)  N=[1]  D="[tau  1]"  Y0=preA  U0=0
      settings: AttributesFormatString=pre-activation: %<Y0>
  Fmax : Gain  Gain=FmaxHAM  SaturateOnIntegerOverflow=on  OutDataTypeStr=Inherit: Same as input  ParamDataTypeStr=Inherit: Same as input
  Fv = Fse / (A*Fce) : Product  Inputs=*/  SaturateOnIntegerOverflow=on  InputSameDT=on  OutDataTypeStr=Inherit: Same as first input
  Integrator : Integrator  InitialConditionSource=external  LowerSaturationLimit=0.05
  PE force-length relation : Subsystem
  SE force-length relation : Subsystem
  Saturation : Saturate  UpperLimit=1  LowerLimit=0.01
  Sum : Sum  Inputs=|+-  SaturateOnIntegerOverflow=on  InputSameDT=on  OutDataTypeStr=Inherit: Same as first input
  Sum2 : Sum  Inputs=|-+  SaturateOnIntegerOverflow=on  InputSameDT=on  OutDataTypeStr=Inherit: Same as first input
  Sum3 : Sum  SaturateOnIntegerOverflow=on  InputSameDT=on  OutDataTypeStr=Inherit: Same as first input
  Sum4 : Sum  SaturateOnIntegerOverflow=on  InputSameDT=on  OutDataTypeStr=Inherit: Same as first input
  lce/lopt : Gain  Gain=1/loptHAM  SaturateOnIntegerOverflow=on  OutDataTypeStr=Inherit: Same as input  ParamDataTypeStr=Inherit: Same as input
  vmax*lopt : Gain  Gain=vmaxHAM*loptHAM  SaturateOnIntegerOverflow=on  OutDataTypeStr=Inherit: Same as input  ParamDataTypeStr=Inherit: Same as input
  Fmtc : Outport  InitialOutput=0
  Lce : Outport  Port=2  InitialOutput=0
  Vce : Outport  Port=3  InitialOutput=0
  A : Outport  Port=4  InitialOutput=0
  wires:
  Integrator/1 -> Sum/2, lce/lopt/1, Lce/1  "lce"
  Sum/1 -> 1/lslack/1  "lse"
  lce/lopt/1 -> CE force-length relation/1(lce [lopt]), BE force-length relation/1(lce [lopt]), PE force-length relation/1(lce [lopt])
  Fv = Fse / (A*Fce)/1 -> CE inverse force-velocity relation/1(Fv[Fmax])  "fv"
  vmax*lopt/1 -> Integrator/1, Vce/1  "vce"
  lmtc [m]/1 -> Sum2/2, Sum/1  "lmtc"
  Fmax/1 -> Fmtc/1  "Fmtc"
  1/lslack/1 -> SE force-length relation/1(lse [lslack])
  SE force-length relation/1(fse [Fmax]) -> Fmax/1, Sum4/1
  Sum2/1 -> Integrator/2
  Constant/1 -> Sum2/1
  CE force-length relation/1(fce [Fmax]) -> 1/1
  Sum4/1 -> Fv = Fse / (A*Fce)/1
  PE force-length relation/1(fpe [Fmax]) -> Sum3/1
  1/1 -> Sum3/2
  BE force-length relation/1(fbe [Fmax]) -> Sum4/2
  Sum3/1 -> Fv = Fse / (A*Fce)/2
  CE inverse force-velocity relation/1(v[vmax]) -> vmax*lopt/1
  STIM/1 -> ECC TransferFcn/1
  ECC TransferFcn/1 -> Saturation/1
  Saturation/1 -> 1/2, A/1

== system ATRIAS_vnmc/control/Virtual Neuromuscular Control/Muscle Layer/HAM Link ==
  note: HAM Attachment
  phi34 [rad] : Inport
  phi23 [rad] : Inport  Port=2
  Constant1 : Constant  Value=rHAMk
  Constant2 : Constant  Value=phirefHAMk
  Constant3 : Constant  Value=rHAMh
  Constant4 : Constant  Value=lslackHAM+loptHAM
  Constant5 : Constant  Value=phirefHAMh
  Gain2 : Gain  Gain=rhoHAMh
  Gain4 : Gain  Gain=rhoHAMk
  Product : Product  RndMeth=Zero
  Product1 : Product  RndMeth=Zero
  Sum1 : Sum  Inputs=|+-
  Sum4 : Sum  Inputs=|+-
  Sum5 : Sum  Inputs=-++
  lmtu [m] : Outport
  lever34 [m] : Outport  Port=2
  lever23 [m] : Outport  Port=3
  wires:
  Sum5/1 -> lmtu [m]/1
  Constant4/1 -> Sum5/2
  Gain4/1 -> Sum5/3
  Gain2/1 -> Sum5/1
  phi34 [rad]/1 -> Sum4/1
  Constant5/1 -> Sum4/2
  Sum4/1 -> Product/1
  Constant3/1 -> Product/2, lever34 [m]/1
  Product/1 -> Gain2/1
  phi23 [rad]/1 -> Sum1/1
  Constant2/1 -> Sum1/2
  Sum1/1 -> Product1/1
  Constant1/1 -> Product1/2, lever23 [m]/1
  Product1/1 -> Gain4/1

== system ATRIAS_vnmc/control/Virtual Neuromuscular Control/Muscle Layer/HAM Link1 ==
  note: HAM Attachment
  phi34 [rad] : Inport
  phi23 [rad] : Inport  Port=2
  Constant1 : Constant  Value=rHAMk
  Constant2 : Constant  Value=phirefHAMk
  Constant3 : Constant  Value=rHAMh
  Constant4 : Constant  Value=lslackHAM+loptHAM
  Constant5 : Constant  Value=phirefHAMh
  Gain2 : Gain  Gain=rhoHAMh
  Gain4 : Gain  Gain=rhoHAMk
  Product : Product  RndMeth=Zero
  Product1 : Product  RndMeth=Zero
  Sum1 : Sum  Inputs=|+-
  Sum4 : Sum  Inputs=|+-
  Sum5 : Sum  Inputs=-++
  lmtu [m] : Outport
  lever34 [m] : Outport  Port=2
  lever23 [m] : Outport  Port=3
  wires:
  Sum5/1 -> lmtu [m]/1
  Constant4/1 -> Sum5/2
  Gain4/1 -> Sum5/3
  Gain2/1 -> Sum5/1
  phi34 [rad]/1 -> Sum4/1
  Constant5/1 -> Sum4/2
  Sum4/1 -> Product/1
  Constant3/1 -> Product/2, lever34 [m]/1
  Product/1 -> Gain2/1
  phi23 [rad]/1 -> Sum1/1
  Constant2/1 -> Sum1/2
  Sum1/1 -> Product1/1
  Constant1/1 -> Product1/2, lever23 [m]/1
  Product1/1 -> Gain4/1

== system ATRIAS_vnmc/control/Virtual Neuromuscular Control/Muscle Layer/HAM1 ==
  note: SOLEUS Muscle-Tendon Dynamics
  note: Excitation Contraction Coupling
  STIM : Inport
  lmtc [m] : Inport  Port=2
  1 : Product  Inputs=**  SaturateOnIntegerOverflow=on  InputSameDT=on  OutDataTypeStr=Inherit: Same as first input
  1/lslack : Gain  Gain=1/lslackHAM  SaturateOnIntegerOverflow=on  OutDataTypeStr=Inherit: Same as input  ParamDataTypeStr=Inherit: Same as input
  BE force-length relation : Subsystem
  CE force-length relation : Subsystem
  CE inverse force-velocity relation : Subsystem
  Constant : Constant  Value=lslackHAM
  ECC TransferFcn : simulink_extras/Additional Linear/Transfer Fcn (with initial outputs)  N=[1]  D="[tau  1]"  Y0=preA  U0=0
      settings: AttributesFormatString=pre-activation: %<Y0>
  Fmax : Gain  Gain=FmaxHAM  SaturateOnIntegerOverflow=on  OutDataTypeStr=Inherit: Same as input  ParamDataTypeStr=Inherit: Same as input
  Fv = Fse / (A*Fce) : Product  Inputs=*/  SaturateOnIntegerOverflow=on  InputSameDT=on  OutDataTypeStr=Inherit: Same as first input
  Integrator : Integrator  InitialConditionSource=external  LowerSaturationLimit=0.05
  PE force-length relation : Subsystem
  SE force-length relation : Subsystem
  Saturation : Saturate  UpperLimit=1  LowerLimit=0.01
  Sum : Sum  Inputs=|+-  SaturateOnIntegerOverflow=on  InputSameDT=on  OutDataTypeStr=Inherit: Same as first input
  Sum2 : Sum  Inputs=|-+  SaturateOnIntegerOverflow=on  InputSameDT=on  OutDataTypeStr=Inherit: Same as first input
  Sum3 : Sum  SaturateOnIntegerOverflow=on  InputSameDT=on  OutDataTypeStr=Inherit: Same as first input
  Sum4 : Sum  SaturateOnIntegerOverflow=on  InputSameDT=on  OutDataTypeStr=Inherit: Same as first input
  lce/lopt : Gain  Gain=1/loptHAM  SaturateOnIntegerOverflow=on  OutDataTypeStr=Inherit: Same as input  ParamDataTypeStr=Inherit: Same as input
  vmax*lopt : Gain  Gain=vmaxHAM*loptHAM  SaturateOnIntegerOverflow=on  OutDataTypeStr=Inherit: Same as input  ParamDataTypeStr=Inherit: Same as input
  Fmtc : Outport  InitialOutput=0
  Lce : Outport  Port=2  InitialOutput=0
  Vce : Outport  Port=3  InitialOutput=0
  A : Outport  Port=4  InitialOutput=0
  wires:
  Integrator/1 -> Sum/2, lce/lopt/1, Lce/1  "lce"
  Sum/1 -> 1/lslack/1  "lse"
  lce/lopt/1 -> CE force-length relation/1(lce [lopt]), BE force-length relation/1(lce [lopt]), PE force-length relation/1(lce [lopt])
  Fv = Fse / (A*Fce)/1 -> CE inverse force-velocity relation/1(Fv[Fmax])  "fv"
  vmax*lopt/1 -> Integrator/1, Vce/1  "vce"
  lmtc [m]/1 -> Sum2/2, Sum/1  "lmtc"
  Fmax/1 -> Fmtc/1  "Fmtc"
  1/lslack/1 -> SE force-length relation/1(lse [lslack])
  SE force-length relation/1(fse [Fmax]) -> Fmax/1, Sum4/1
  Sum2/1 -> Integrator/2
  Constant/1 -> Sum2/1
  CE force-length relation/1(fce [Fmax]) -> 1/1
  Sum4/1 -> Fv = Fse / (A*Fce)/1
  PE force-length relation/1(fpe [Fmax]) -> Sum3/1
  1/1 -> Sum3/2
  BE force-length relation/1(fbe [Fmax]) -> Sum4/2
  Sum3/1 -> Fv = Fse / (A*Fce)/2
  CE inverse force-velocity relation/1(v[vmax]) -> vmax*lopt/1
  STIM/1 -> ECC TransferFcn/1
  ECC TransferFcn/1 -> Saturation/1
  Saturation/1 -> 1/2, A/1

== system ATRIAS_vnmc/control/Virtual Neuromuscular Control/Muscle Layer/HFL ==
  note: SOLEUS Muscle-Tendon Dynamics
  note: Excitation Contraction Coupling
  STIM : Inport
  lmtc [m] : Inport  Port=2
  1 : Product  Inputs=**  SaturateOnIntegerOverflow=on  InputSameDT=on  OutDataTypeStr=Inherit: Same as first input
  1/lslack : Gain  Gain=1/lslackHFL  SaturateOnIntegerOverflow=on  OutDataTypeStr=Inherit: Same as input  ParamDataTypeStr=Inherit: Same as input
  BE force-length relation : Subsystem
  CE force-length relation : Subsystem
  CE inverse force-velocity relation : Subsystem
  Constant : Constant  Value=lslackHFL
  ECC TransferFcn : simulink_extras/Additional Linear/Transfer Fcn (with initial outputs)  N=[1]  D="[tau  1]"  Y0=preA  U0=0
      settings: AttributesFormatString=pre-activation: %<Y0>
  Fmax : Gain  Gain=FmaxHFL  SaturateOnIntegerOverflow=on  OutDataTypeStr=Inherit: Same as input  ParamDataTypeStr=Inherit: Same as input
  Fv = Fse / (A*Fce) : Product  Inputs=*/  SaturateOnIntegerOverflow=on  InputSameDT=on  OutDataTypeStr=Inherit: Same as first input
  Integrator : Integrator  InitialConditionSource=external  LowerSaturationLimit=0.05
  PE force-length relation : Subsystem
  SE force-length relation : Subsystem
  Saturation : Saturate  UpperLimit=1  LowerLimit=0.01
  Sum : Sum  Inputs=|+-  SaturateOnIntegerOverflow=on  InputSameDT=on  OutDataTypeStr=Inherit: Same as first input
  Sum2 : Sum  Inputs=|-+  SaturateOnIntegerOverflow=on  InputSameDT=on  OutDataTypeStr=Inherit: Same as first input
  Sum3 : Sum  SaturateOnIntegerOverflow=on  InputSameDT=on  OutDataTypeStr=Inherit: Same as first input
  Sum4 : Sum  SaturateOnIntegerOverflow=on  InputSameDT=on  OutDataTypeStr=Inherit: Same as first input
  lce/lopt : Gain  Gain=1/loptHFL  SaturateOnIntegerOverflow=on  OutDataTypeStr=Inherit: Same as input  ParamDataTypeStr=Inherit: Same as input
  vmax*lopt : Gain  Gain=vmaxHFL*loptHFL  SaturateOnIntegerOverflow=on  OutDataTypeStr=Inherit: Same as input  ParamDataTypeStr=Inherit: Same as input
  Fmtc : Outport  InitialOutput=0
  Lce : Outport  Port=2  InitialOutput=0
  Vce : Outport  Port=3  InitialOutput=0
  A : Outport  Port=4  InitialOutput=0
  wires:
  Integrator/1 -> Sum/2, lce/lopt/1, Lce/1  "lce"
  Sum/1 -> 1/lslack/1  "lse"
  lce/lopt/1 -> CE force-length relation/1(lce [lopt]), BE force-length relation/1(lce [lopt]), PE force-length relation/1(lce [lopt])
  Fv = Fse / (A*Fce)/1 -> CE inverse force-velocity relation/1(Fv[Fmax])  "fv"
  vmax*lopt/1 -> Integrator/1, Vce/1  "vce"
  lmtc [m]/1 -> Sum2/2, Sum/1  "lmtc"
  Fmax/1 -> Fmtc/1  "Fmtc"
  1/lslack/1 -> SE force-length relation/1(lse [lslack])
  SE force-length relation/1(fse [Fmax]) -> Fmax/1, Sum4/1
  Sum2/1 -> Integrator/2
  Constant/1 -> Sum2/1
  CE force-length relation/1(fce [Fmax]) -> 1/1
  Sum4/1 -> Fv = Fse / (A*Fce)/1
  PE force-length relation/1(fpe [Fmax]) -> Sum3/1
  1/1 -> Sum3/2
  BE force-length relation/1(fbe [Fmax]) -> Sum4/2
  Sum3/1 -> Fv = Fse / (A*Fce)/2
  CE inverse force-velocity relation/1(v[vmax]) -> vmax*lopt/1
  STIM/1 -> ECC TransferFcn/1
  ECC TransferFcn/1 -> Saturation/1
  Saturation/1 -> A/1, 1/2

== system ATRIAS_vnmc/control/Virtual Neuromuscular Control/Muscle Layer/HFL Link ==
  note: HFL Attachment
  phi34 [rad] : Inport
  Constant : Constant  Value=lslackHFL+loptHFL
  Constant1 : Constant  Value=rHFL
  Constant2 : Constant  Value=phirefHFL
  Gain2 : Gain  Gain=rhoHFL
  Product : Product  RndMeth=Zero
  Sum2 : Sum  Inputs=|+-
  Sum5 : Sum  Inputs=|++
  lmtu [m] : Outport
  lever [m] : Outport  Port=2
  wires:
  Constant/1 -> Sum5/1
  Sum5/1 -> lmtu [m]/1
  Product/1 -> Gain2/1
  phi34 [rad]/1 -> Sum2/1
  Constant2/1 -> Sum2/2
  Sum2/1 -> Product/1
  Constant1/1 -> Product/2, lever [m]/1
  Gain2/1 -> Sum5/2
